simulink model "pulScope"  (R2023b)
settings: Solver=VariableStepAuto  StartTime=0.0  StopTime=10.0  RelTol=1e-3
settings Model: Creator=mhagh  LastModifiedBy=mhagh

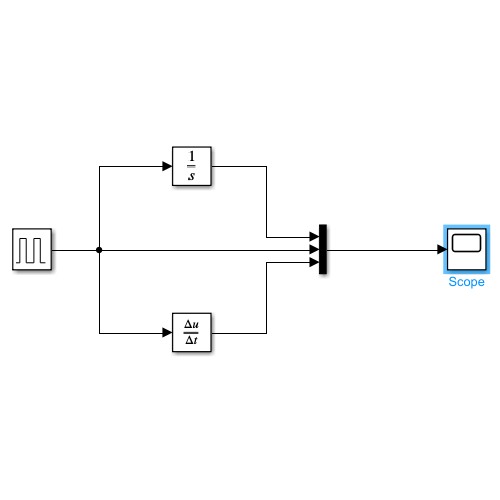
[thumbnail: Simulink's stored preview of the top-level diagram]
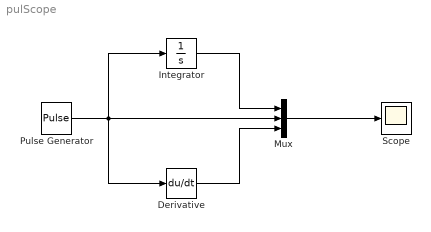
== system pulScope ==
  Derivative : Derivative
  Integrator : Integrator
  Mux : Mux  Inputs=3
  Pulse Generator : DiscretePulseGenerator  PulseType=Time based  Period=10  PulseWidth=5
  Scope : Scope
  wires:
  Pulse Generator/1 -> Mux/2, Derivative/1, Integrator/1
  Integrator/1 -> Mux/1
  Mux/1 -> Scope/1
  Derivative/1 -> Mux/3
